simulink model "six_plus_six_AcmsteeringV09_main"  (R2014a)
settings: Solver=FixedStepDiscrete  StartTime=0.0  StopTime=10.0  FixedStep=0.0005  RelTol=1e-3
InitFcn:
  | Veh_Par_wxt
values from neighbouring files (symbols this model uses):
  acc_spdctl = [0 100]    [Veh_Par_wxt.m]
  ag_thr = ecucoder_cal(ag_thr)    [Veh_Par_wxt.m]
  B = 1.8    [Veh_Par_wxt.m]
  bra_em = 100    [Veh_Par_wxt.m]
  bra_pre_gz2 = 100/3    (= 33.3333333333)    [Veh_Par_wxt.m]
  bra_pre_gz34 = 10/3    (= 3.33333333333)    [Veh_Par_wxt.m]
  bra_pre_yd = 10/2    (= 5)    [Veh_Par_wxt.m]
  brakepre_dem_data = [0 1 2 3 4 5 6 7 8 9 10]    [Veh_Par_wxt.m]
  brakeTrq_dem_data = [0 125 251 376 502 627 753 878 1004 1129 1255]    [Veh_Par_wxt.m]
  bratrq_max = 4*1255    (= 5020)    [Veh_Par_wxt.m]
  eff_tran = 0.9    [Veh_Par_wxt.m]
  ESP_switch = ecucoder_cal(ESP_switch)    [Veh_Par_wxt.m]
  G = Mass*g    (= 15696)    [Veh_Par_wxt.m]
  kd1 = ecucoder_cal(kd1)    [Veh_Par_wxt.m]
  kd2 = 0    [Veh_Par_wxt.m]
  ki1 = ecucoder_cal(ki1)    [Veh_Par_wxt.m]
  ki2 = 1    [Veh_Par_wxt.m]
  kp1 = ecucoder_cal(kp1)    [Veh_Par_wxt.m]
  kp2 = 300    [Veh_Par_wxt.m]
  L = L1+L2    (= 2.9)    [Veh_Par_wxt.m]
  premax = 100    [Veh_Par_wxt.m]
  Radius = 0.4572/2    (= 0.2286)    [Veh_Par_wxt.m]
  RC_switch = ecucoder_cal(RC_switch)    [Veh_Par_wxt.m]
  s_opt_yi = 0.15    [Veh_Par_wxt.m]
  s_opt_zhuan = 0.8    [Veh_Par_wxt.m]
  s_opt_zhuan_add = 0.05    [Veh_Par_wxt.m]
  s_opt_zhuan_table = [0.8 0.8 0.3 0.3]    [Veh_Par_wxt.m]
  spd_map_mot = [0 499.85 999.79 1500 2000 2500 3000 3500 4000 4500 4999.8 5999.8]    [Veh_Par_wxt.m]
  spd_spdctl = [0 500]    [Veh_Par_wxt.m]
  speed_thr_park = 5/3.6/Radius*tras_ratio*30/pi    (= 464.143899364)    [Veh_Par_wxt.m]
  TCS_switch = ecucoder_cal(TCS_switch)    [Veh_Par_wxt.m]
  tras_ratio = 8    [Veh_Par_wxt.m]
  trq_map_mot = [70.5 70.012 71.154 65.797 53.917 45.159 38.073 32.685 27.48 17.133 14.949 10.07]    [Veh_Par_wxt.m]
  trqmax_yd = 70.5    [Veh_Par_wxt.m]
  trqmax_zx = 70.5    [Veh_Par_wxt.m]
  trqmaxneg = -70.5    [Veh_Par_wxt.m]
  v_gain = 0.9    [Veh_Par_wxt.m]
  v_table = [0 5 20 100]    [Veh_Par_wxt.m]
  v_thr_park = 5    [Veh_Par_wxt.m]
  zhidong_bianmazhi = [-140000 750000]    [Veh_Par_wxt.m]
  zhidong_down = -140000    [Veh_Par_wxt.m]
  zhidong_up = 750000    [Veh_Par_wxt.m]
  zhidong_youmen = [0 100]    [Veh_Par_wxt.m]
  zhuanxiang_bianmazhi = [-400000 0 400000]    [Veh_Par_wxt.m]
  zhuanxiang_down = -400000    [Veh_Par_wxt.m]
  zhuanxiang_up = 400000    [Veh_Par_wxt.m]
  zhuanxiang_youmen = [-100 0 100]    [Veh_Par_wxt.m]
undefined symbols (not defined in the file or in its folder): ecucoder_acal, guzhang_lf, guzhang_lm, guzhang_lr, guzhang_rf, guzhang_rm, guzhang_rr, myFIS
libraries: simulink x979, ec5744lib x59, fuzblock x2
(part 23 of 26)

== matlab function six_plus_six_AcmsteeringV09_main/MainControl/mode_control/backward/backward/Drive/容错控制/MATLAB Function ==
  data: trq_dem_l input; trq_dem_lf output; trq_dem_lm output; trq_dem_r input; trqlim_lf input; trqlim_lm input; trqlim_lr input; trqlim_rf input; trqlim_rm input; trqlim_rr input; guzhang_lf input; guzhang_lm input; guzhang_lr input; guzhang_rf input; guzhang_rm input; guzhang_rr input; trq_dem_lr output; trq_dem_rf output; trq_dem_rm output; trq_dem_rr output; bra_pre_l output; bra_pre_r output; bra_pre_gz2 input; bra_pre_gz34 input; mode output int8
function [trq_dem_lf,trq_dem_lm,trq_dem_lr,trq_dem_rf,trq_dem_rm,trq_dem_rr,bra_pre_l,bra_pre_r,mode] = fcn(trq_dem_l,trq_dem_r,trqlim_lf,trqlim_lm,trqlim_lr,trqlim_rf,trqlim_rm,trqlim_rr,guzhang_lf,guzhang_lm,guzhang_lr,guzhang_rf,guzhang_rm,guzhang_rr,bra_pre_gz2,bra_pre_gz34)
%#codegen
if guzhang_lf==0 && guzhang_lm==0 && guzhang_lr==0 && guzhang_rf==0 && guzhang_rm==0 && guzhang_rr==0    %0电机故障,平均分配
    trq_dem_lf=single(trq_dem_l/3);
    trq_dem_lm=single(trq_dem_l/3);
    trq_dem_lr=single(trq_dem_l/3);
    trq_dem_rf=single(trq_dem_r/3);
    trq_dem_rm=single(trq_dem_r/3);
    trq_dem_rr=single(trq_dem_r/3);
    bra_pre_l=single(0);
    bra_pre_r=single(0);
    mode=int8(1);
    
    
    
    
elseif guzhang_lf==1 && guzhang_lm==0 && guzhang_lr==0 && guzhang_rf==0 && guzhang_rm==0 && guzhang_rr==0    %1电机故障，同侧电机进行力矩转移，超过限值后，对侧亦降扭。  左前
    trq_dem_lf=single(0);
    trq_dem_lm=single(min(trq_dem_l/2,trqlim_lm));
    trq_dem_lr=single(min(trq_dem_l/2,trqlim_lr));
    trq_dem_rf=single((trq_dem_r-(trq_dem_l-trq_dem_lm-trq_dem_lr))/3);
    trq_dem_rm=single((trq_dem_r-(trq_dem_l-trq_dem_lm-trq_dem_lr))/3);
    trq_dem_rr=single((trq_dem_r-(trq_dem_l-trq_dem_lm-trq_dem_lr))/3);
    bra_pre_l=single(0);
    bra_pre_r=single(0);
    mode=int8(2);
elseif guzhang_lf==0 && guzhang_lm==1 && guzhang_lr==0 && guzhang_rf==0 && guzhang_rm==0 && guzhang_rr==0    %1电机故障，同侧电机进行力矩转移，超过限值后，对侧亦降扭。 左中
    trq_dem_lf=single(min(trq_dem_l/2,trqlim_lf));
    trq_dem_lm=single(0);
    trq_dem_lr=single(min(trq_dem_l/2,trqlim_lr));
    trq_dem_rf=single((trq_dem_r-(trq_dem_l-trq_dem_lf-trq_dem_lr))/3);
    trq_dem_rm=single((trq_dem_r-(trq_dem_l-trq_dem_lf-trq_dem_lr))/3);
    trq_dem_rr=single((trq_dem_r-(trq_dem_l-trq_dem_lf-trq_dem_lr))/3);
    bra_pre_l=single(0);
    bra_pre_r=single(0);
    mode=int8(3);
elseif guzhang_lf==0 && guzhang_lm==0 && guzhang_lr==1 && guzhang_rf==0 && guzhang_rm==0 && guzhang_rr==0    %1电机故障，同侧电机进行力矩转移，超过限值后，对侧亦降扭。 左后
    trq_dem_lf=single(min(trq_dem_l/2,trqlim_lf));
    trq_dem_lm=single(min(trq_dem_l/2,trqlim_lm));
    trq_dem_lr=single(0);
    trq_dem_rf=single((trq_dem_r-(trq_dem_l-trq_dem_lf-trq_dem_lm))/3);
    trq_dem_rm=single((trq_dem_r-(trq_dem_l-trq_dem_lf-trq_dem_lm))/3);
    trq_dem_rr=single((trq_dem_r-(trq_dem_l-trq_dem_lf-trq_dem_lm))/3);
    bra_pre_l=single(0);
    bra_pre_r=single(0);
    mode=int8(4);
elseif guzhang_lf==0 && guzhang_lm==0 && guzhang_lr==0 && guzhang_rf==1 && guzhang_rm==0 && guzhang_rr==0    %1电机故障，同侧电机进行力矩转移，超过限值后，对侧亦降扭。  右前
    trq_dem_rf=single(0);
    trq_dem_rm=single(min(trq_dem_r/2,trqlim_rm));
    trq_dem_rr=single(min(trq_dem_r/2,trqlim_rr));
    trq_dem_lf=single((trq_dem_l-(trq_dem_r-trq_dem_rm-trq_dem_rr))/3);
    trq_dem_lm=single((trq_dem_l-(trq_dem_r-trq_dem_rm-trq_dem_rr))/3);
    trq_dem_lr=single((trq_dem_l-(trq_dem_r-trq_dem_rm-trq_dem_rr))/3);
    bra_pre_l=single(0);
    bra_pre_r=single(0);
    mode=int8(5);
elseif guzhang_lf==0 && guzhang_lm==0 && guzhang_lr==0 && guzhang_rf==0 && guzhang_rm==1 && guzhang_rr==0    %1电机故障，同侧电机进行力矩转移，超过限值后，对侧亦降扭。 右中
    trq_dem_rf=single(min(trq_dem_r/2,trqlim_rf));
    trq_dem_rm=single(0);
    trq_dem_rr=single(min(trq_dem_r/2,trqlim_rr));
    trq_dem_lf=single((trq_dem_l-(trq_dem_r-trq_dem_rf-trq_dem_rr))/3);
    trq_dem_lm=single((trq_dem_l-(trq_dem_r-trq_dem_rf-trq_dem_rr))/3);
    trq_dem_lr=single((trq_dem_l-(trq_dem_r-trq_dem_rf-trq_dem_rr))/3);
    bra_pre_l=single(0);
    bra_pre_r=single(0);
    mode=int8(6);
elseif guzhang_lf==0 && guzhang_lm==0 && guzhang_lr==0 && guzhang_rf==0 && guzhang_rm==0 && guzhang_rr==1    %1电机故障，同侧电机进行力矩转移，超过限值后，对侧亦降扭。 右后
    trq_dem_rf=single(min(trq_dem_r/2,trqlim_rf));
    trq_dem_rm=single(min(trq_dem_r/2,trqlim_rm));
    trq_dem_rr=single(0);
    trq_dem_lf=single((trq_dem_l-(trq_dem_r-trq_dem_rf-trq_dem_rm))/3);
    trq_dem_lm=single((trq_dem_l-(trq_dem_r-trq_dem_rf-trq_dem_rm))/3);
    trq_dem_lr=single((trq_dem_l-(trq_dem_r-trq_dem_rf-trq_dem_rm))/3);
    bra_pre_l=single(0);
    bra_pre_r=single(0);
    mode=int8(7);
    
    
    
    
    
    
elseif guzhang_lf==1 && guzhang_lm==1 && guzhang_lr==0 && guzhang_rf==0 && guzhang_rm==0 && guzhang_rr==0    %2电机故障，同侧电机进行力矩转移，超过限值后，对侧亦降扭。  左前 左中   左侧
    trq_dem_lf=single(0);
    trq_dem_lm=single(0);
    trq_dem_lr=single(min(trq_dem_l,trqlim_lr));
    trq_dem_rf=single((trq_dem_r-(trq_dem_l-trq_dem_lr))/3);
    trq_dem_rm=single((trq_dem_r-(trq_dem_l-trq_dem_lr))/3);
    trq_dem_rr=single((trq_dem_r-(trq_dem_l-trq_dem_lr))/3);
    bra_pre_l=single(0);
    bra_pre_r=single(0);
    mode=int8(8);
elseif guzhang_lf==1 && guzhang_lm==0 && guzhang_lr==1 && guzhang_rf==0 && guzhang_rm==0 && guzhang_rr==0    %2电机故障，同侧电机进行力矩转移，超过限值后，对侧亦降扭。  左前 左后
    trq_dem_lf=single(0);
    trq_dem_lm=single(min(trq_dem_l,trqlim_lm));
    trq_dem_lr=single(0);
    trq_dem_rf=single((trq_dem_r-(trq_dem_l-trq_dem_lm))/3);
    trq_dem_rm=single((trq_dem_r-(trq_dem_l-trq_dem_lm))/3);
    trq_dem_rr=single((trq_dem_r-(trq_dem_l-trq_dem_lm))/3);
    bra_pre_l=single(0);
    bra_pre_r=single(0);
    mode=int8(9);
elseif guzhang_lf==0 && guzhang_lm==1 && guzhang_lr==1 && guzhang_rf==0 && guzhang_rm==0 && guzhang_rr==0    %2电机故障，同侧电机进行力矩转移，超过限值后，对侧亦降扭。  左中 左后
    trq_dem_lf=single(min(trq_dem_l,trqlim_lf));
    trq_dem_lm=single(0);
    trq_dem_lr=single(0);
    trq_dem_rf=single((trq_dem_r-(trq_dem_l-trq_dem_lf))/3);
    trq_dem_rm=single((trq_dem_r-(trq_dem_l-trq_dem_lf))/3);
    trq_dem_rr=single((trq_dem_r-(trq_dem_l-trq_dem_lf))/3);
    bra_pre_l=single(0);
    bra_pre_r=single(0);
    mode=int8(10);
    
elseif guzhang_lf==0 && guzhang_lm==0 && guzhang_lr==0 && guzhang_rf==1 && guzhang_rm==1 && guzhang_rr==0    %2电机故障，同侧电机进行力矩转移，超过限值后，对侧亦降扭。  右前 右中   右侧
    trq_dem_rf=single(0);
    trq_dem_rm=single(0);
    trq_dem_rr=single(min(trq_dem_r,trqlim_rr));
    trq_dem_lf=single((trq_dem_l-(trq_dem_r-trq_dem_rr))/3);
    trq_dem_lm=single((trq_dem_l-(trq_dem_r-trq_dem_rr))/3);
    trq_dem_lr=single((trq_dem_l-(trq_dem_r-trq_dem_rr))/3);
    bra_pre_l=single(0);
    bra_pre_r=single(0);
    mode=int8(11);
elseif guzhang_lf==0 && guzhang_lm==0 && guzhang_lr==0 && guzhang_rf==1 && guzhang_rm==0 && guzhang_rr==1    %2电机故障，同侧电机进行力矩转移，超过限值后，对侧亦降扭。  右前 右后
    trq_dem_rf=single(0);
    trq_dem_rm=single(min(trq_dem_r,trqlim_rm));
    trq_dem_rr=single(0);
    trq_dem_lf=single((trq_dem_l-(trq_dem_r-trq_dem_rm))/3);
    trq_dem_lm=single((trq_dem_l-(trq_dem_r-trq_dem_rm))/3);
    trq_dem_lr=single((trq_dem_l-(trq_dem_r-trq_dem_rm))/3);
    bra_pre_l=single(0);
    bra_pre_r=single(0);
    mode=int8(12);
elseif guzhang_lf==0 && guzhang_lm==0 && guzhang_lr==0 && guzhang_rf==0 && guzhang_rm==1 && guzhang_rr==1    %2电机故障，同侧电机进行力矩转移，超过限值后，对侧亦降扭。  右中 右后
    trq_dem_rf=single(min(trq_dem_r,trqlim_rf));
    trq_dem_rm=single(0);
    trq_dem_rr=single(0);
    trq_dem_lf=single((trq_dem_l-(trq_dem_r-trq_dem_rf))/3);
    trq_dem_lm=single((trq_dem_l-(trq_dem_r-trq_dem_rf))/3);
    trq_dem_lr=single((trq_dem_l-(trq_dem_r-trq_dem_rf))/3);
    bra_pre_l=single(0);
    bra_pre_r=single(0);
    mode=int8(13);
    
elseif guzhang_lf==1 && guzhang_lm==0 && guzhang_lr==0 && guzhang_rf==1 && guzhang_rm==0 && guzhang_rr==0    %2电机故障，同侧电机进行力矩转移，超过限值后，对侧亦降扭。  左前-右前 对侧
    trq_dem_lf=single(0);
    trq_dem_rf=single(0);
    trq_dem_lm=single(min(trq_dem_l/2,trqlim_lm));
    trq_dem_lr=single(min(trq_dem_l/2,trqlim_lr));
    trq_dem_rm=single(min(trq_dem_r/2,trqlim_rm));
    trq_dem_rr=single(min(trq_dem_r/2,trqlim_rr));
    if (trq_dem_l-trq_dem_lm-trq_dem_lr)>=(trq_dem_r-trq_dem_rm-trq_dem_rr)
        trq_dem_rm=single(min(trqlim_rm,(trq_dem_r-(trq_dem_l-trq_dem_lm-trq_dem_lr))/2));
        trq_dem_rr=single(min(trqlim_rr,(trq_dem_r-(trq_dem_l-trq_dem_lm-trq_dem_lr))/2));
    else
        trq_dem_lm=single(min(trqlim_lm,(trq_dem_l-(trq_dem_r-trq_dem_rm-trq_dem_rr))/2));
        trq_dem_lr=single(min(trqlim_lr,(trq_dem_l-(trq_dem_r-trq_dem_rm-trq_dem_rr))/2));
    end
    bra_pre_l=single(0);
    bra_pre_r=single(0);
    mode=int8(14);
elseif guzhang_lf==1 && guzhang_lm==0 && guzhang_lr==0 && guzhang_rf==0 && guzhang_rm==1 && guzhang_rr==0    %2电机故障，同侧电机进行力矩转移，超过限值后，对侧亦降扭。  左前-右中
    trq_dem_lf=single(0);
    trq_dem_rm=single(0);
    trq_dem_lm=single(min(trq_dem_l/2,trqlim_lm));
    trq_dem_lr=single(min(trq_dem_l/2,trqlim_lr));
    trq_dem_rf=single(min(trq_dem_r/2,trqlim_rf));
    trq_dem_rr=single(min(trq_dem_r/2,trqlim_rr));
    if (trq_dem_l-trq_dem_lm-trq_dem_lr)>=(trq_dem_r-trq_dem_rf-trq_dem_rr)
        trq_dem_rf=single(min(trqlim_rf,(trq_dem_r-(trq_dem_l-trq_dem_lm-trq_dem_lr))/2));
        trq_dem_rr=single(min(trqlim_rr,(trq_dem_r-(trq_dem_l-trq_dem_lm-trq_dem_lr))/2));
    else
        trq_dem_lm=single(min(trqlim_lm,(trq_dem_l-(trq_dem_r-trq_dem_rf-trq_dem_rr))/2));
        trq_dem_lr=single(min(trqlim_lr,(trq_dem_l-(trq_dem_r-trq_dem_rf-trq_dem_rr))/2));
    end
    bra_pre_l=single(0);
    bra_pre_r=single(0);
    mode=int8(15);
elseif guzhang_lf==1 && guzhang_lm==0 && guzhang_lr==0 && guzhang_rf==0 && guzhang_rm==0 && guzhang_rr==1    %2电机故障，同侧电机进行力矩转移，超过限值后，对侧亦降扭。  左前-右后
    trq_dem_lf=single(0);
    trq_dem_rr=single(0);
    trq_dem_lm=single(min(trq_dem_l/2,trqlim_lm));
    trq_dem_lr=single(min(trq_dem_l/2,trqlim_lr));
    trq_dem_rf=single(min(trq_dem_r/2,trqlim_rf));
    trq_dem_rm=single(min(trq_dem_r/2,trqlim_rm));
    if (trq_dem_l-trq_dem_lm-trq_dem_lr)>=(trq_dem_r-trq_dem_rf-trq_dem_rm)
        trq_dem_rf=single(min(trqlim_rf,(trq_dem_r-(trq_dem_l-trq_dem_lm-trq_dem_lr))/2));
        trq_dem_rm=single(min(trqlim_rm,(trq_dem_r-(trq_dem_l-trq_dem_lm-trq_dem_lr))/2));
    else
        trq_dem_lm=single(min(trqlim_lm,(trq_dem_l-(trq_dem_r-trq_dem_rf-trq_dem_rm))/2));
        trq_dem_lr=single(min(trqlim_lr,(trq_dem_l-(trq_dem_r-trq_dem_rf-trq_dem_rm))/2));
    end
    bra_pre_l=single(0);
    bra_pre_r=single(0);
    mode=int8(16);
    
elseif guzhang_lf==0 && guzhang_lm==1 && guzhang_lr==0 && guzhang_rf==1 && guzhang_rm==0 && guzhang_rr==0    %2电机故障，同侧电机进行力矩转移，超过限值后，对侧亦降扭。  左中-右前
    trq_dem_lm=single(0);
    trq_dem_rf=single(0);
    trq_dem_lf=single(min(trq_dem_l/2,trqlim_lf));
    trq_dem_lr=single(min(trq_dem_l/2,trqlim_lr));
    trq_dem_rm=single(min(trq_dem_r/2,trqlim_rm));
    trq_dem_rr=single(min(trq_dem_r/2,trqlim_rr));
    if (trq_dem_l-trq_dem_lf-trq_dem_lr)>=(trq_dem_r-trq_dem_rm-trq_dem_rr)
        trq_dem_rm=single(min(trqlim_rm,(trq_dem_r-(trq_dem_l-trq_dem_lf-trq_dem_lr))/2));
        trq_dem_rr=single(min(trqlim_rr,(trq_dem_r-(trq_dem_l-trq_dem_lf-trq_dem_lr))/2));
    else
        trq_dem_lf=single(min(trqlim_lf,(trq_dem_l-(trq_dem_r-trq_dem_rm-trq_dem_rr))/2));
        trq_dem_lr=single(min(trqlim_lr,(trq_dem_l-(trq_dem_r-trq_dem_rm-trq_dem_rr))/2));
    end
    bra_pre_l=single(0);
    bra_pre_r=single(0);
    mode=int8(17);
elseif guzhang_lf==0 && guzhang_lm==1 && guzhang_lr==0 && guzhang_rf==0 && guzhang_rm==1 && guzhang_rr==0    %2电机故障，同侧电机进行力矩转移，超过限值后，对侧亦降扭。  左中-右中
    trq_dem_lm=single(0);
    trq_dem_rm=single(0);
    trq_dem_lf=single(min(trq_dem_l/2,trqlim_lf));
    trq_dem_lr=single(min(trq_dem_l/2,trqlim_lr));
    trq_dem_rf=single(min(trq_dem_r/2,trqlim_rf));
    trq_dem_rr=single(min(trq_dem_r/2,trqlim_rr));
    if (trq_dem_l-trq_dem_lf-trq_dem_lr)>=(trq_dem_r-trq_dem_rf-trq_dem_rr)
        trq_dem_rf=single(min(trqlim_rf,(trq_dem_r-(trq_dem_l-trq_dem_lf-trq_dem_lr))/2));
        trq_dem_rr=single(min(trqlim_rr,(trq_dem_r-(trq_dem_l-trq_dem_lf-trq_dem_lr))/2));
    else
        trq_dem_lf=single(min(trqlim_lf,(trq_dem_l-(trq_dem_r-trq_dem_rf-trq_dem_rr))/2));
        trq_dem_lr=single(min(trqlim_lr,(trq_dem_l-(trq_dem_r-trq_dem_rf-trq_dem_rr))/2));
    end
    bra_pre_l=single(0);
    bra_pre_r=single(0);
    mode=int8(18);
elseif guzhang_lf==0 && guzhang_lm==1 && guzhang_lr==0 && guzhang_rf==0 && guzhang_rm==0 && guzhang_rr==1    %2电机故障，同侧电机进行力矩转移，超过限值后，对侧亦降扭。  左中-右后
    trq_dem_lm=single(0);
    trq_dem_rr=single(0);
    trq_dem_lf=single(min(trq_dem_l/2,trqlim_lf));
    trq_dem_lr=single(min(trq_dem_l/2,trqlim_lr));
    trq_dem_rf=single(min(trq_dem_r/2,trqlim_rf));
    trq_dem_rm=single(min(trq_dem_r/2,trqlim_rm));
    if (trq_dem_l-trq_dem_lf-trq_dem_lr)>=(trq_dem_r-trq_dem_rf-trq_dem_rm)
        trq_dem_rf=single(min(trqlim_rf,(trq_dem_r-(trq_dem_l-trq_dem_lf-trq_dem_lr))/2));
        trq_dem_rm=single(min(trqlim_rm,(trq_dem_r-(trq_dem_l-trq_dem_lf-trq_dem_lr))/2));
    else
        trq_dem_lf=single(min(trqlim_lf,(trq_dem_l-(trq_dem_r-trq_dem_rf-trq_dem_rm))/2));
        trq_dem_lr=single(min(trqlim_lr,(trq_dem_l-(trq_dem_r-trq_dem_rf-trq_dem_rm))/2));
    end
    bra_pre_l=single(0);
    bra_pre_r=single(0);
    mode=int8(19);
    
elseif guzhang_lf==0 && guzhang_lm==0 && guzhang_lr==1 && guzhang_rf==1 && guzhang_rm==0 && guzhang_rr==0    %2电机故障，同侧电机进行力矩转移，超过限值后，对侧亦降扭。  左后-右前
    trq_dem_lr=single(0);
    trq_dem_rf=single(0);
    trq_dem_lf=single(min(trq_dem_l/2,trqlim_lf));
    trq_dem_lm=single(min(trq_dem_l/2,trqlim_lm));
    trq_dem_rm=single(min(trq_dem_r/2,trqlim_rm));
    trq_dem_rr=single(min(trq_dem_r/2,trqlim_rr));
    if (trq_dem_l-trq_dem_lf-trq_dem_lm)>=(trq_dem_r-trq_dem_rm-trq_dem_rr)
        trq_dem_rm=single(min(trqlim_rm,(trq_dem_r-(trq_dem_l-trq_dem_lf-trq_dem_lm))/2));
        trq_dem_rr=single(min(trqlim_rr,(trq_dem_r-(trq_dem_l-trq_dem_lf-trq_dem_lm))/2));
    else
        trq_dem_lf=single(min(trqlim_lf,(trq_dem_l-(trq_dem_r-trq_dem_rm-trq_dem_rr))/2));
        trq_dem_lm=single(min(trqlim_lm,(trq_dem_l-(trq_dem_r-trq_dem_rm-trq_dem_rr))/2));
    end
    bra_pre_l=single(0);
    bra_pre_r=single(0);
    mode=int8(20);
elseif guzhang_lf==0 && guzhang_lm==0 && guzhang_lr==1 && guzhang_rf==0 && guzhang_rm==1 && guzhang_rr==0    %2电机故障，同侧电机进行力矩转移，超过限值后，对侧亦降扭。  左后-右中
    trq_dem_lr=single(0);
    trq_dem_rm=single(0);
    trq_dem_lf=single(min(trq_dem_l/2,trqlim_lf));
    trq_dem_lm=single(min(trq_dem_l/2,trqlim_lm));
    trq_dem_rf=single(min(trq_dem_r/2,trqlim_rf));
    trq_dem_rr=single(min(trq_dem_r/2,trqlim_rr));
    if (trq_dem_l-trq_dem_lf-trq_dem_lm)>=(trq_dem_r-trq_dem_rf-trq_dem_rr)
        trq_dem_rf=single(min(trqlim_rf,(trq_dem_r-(trq_dem_l-trq_dem_lf-trq_dem_lm))/2));
        trq_dem_rr=single(min(trqlim_rr,(trq_dem_r-(trq_dem_l-trq_dem_lf-trq_dem_lm))/2));
    else
        trq_dem_lf=single(min(trqlim_lf,(trq_dem_l-(trq_dem_r-trq_dem_rf-trq_dem_rr))/2));
        trq_dem_lm=single(min(trqlim_lm,(trq_dem_l-(trq_dem_r-trq_dem_rf-trq_dem_rr))/2));
    end
    bra_pre_l=single(0);
    bra_pre_r=single(0);
    mode=int8(21);
elseif guzhang_lf==0 && guzhang_lm==0 && guzhang_lr==1 && guzhang_rf==0 && guzhang_rm==0 && guzhang_rr==1    %2电机故障，同侧电机进行力矩转移，超过限值后，对侧亦降扭。  左后-右后
    trq_dem_lr=single(0);
    trq_dem_rr=single(0);
    trq_dem_lf=single(min(trq_dem_l/2,trqlim_lf));
    trq_dem_lm=single(min(trq_dem_l/2,trqlim_lm));
    trq_dem_rf=single(min(trq_dem_r/2,trqlim_rf));
    trq_dem_rm=single(min(trq_dem_r/2,trqlim_rm));
    if (trq_dem_l-trq_dem_lf-trq_dem_lm)>=(trq_dem_r-trq_dem_rf-trq_dem_rm)
        trq_dem_rf=single(min(trqlim_rf,(trq_dem_r-(trq_dem_l-trq_dem_lf-trq_dem_lm))/2));
        trq_dem_rm=single(min(trqlim_rm,(trq_dem_r-(trq_dem_l-trq_dem_lf-trq_dem_lm))/2));
    else
        trq_dem_lf=single(min(trqlim_lf,(trq_dem_l-(trq_dem_r-trq_dem_rf-trq_dem_rm))/2));
        trq_dem_lm=single(min(trqlim_lm,(trq_dem_l-(trq_dem_r-trq_dem_rf-trq_dem_rm))/2));
    end
    bra_pre_l=single(0);
    bra_pre_r=single(0);
    mode=int8(22);
    
    
    
    
    
    
    
    
    
elseif guzhang_lf==1 && guzhang_lm==1 && guzhang_lr==1 && guzhang_rf==0 && guzhang_rm==0 && guzhang_rr==0    %3电机故障，同侧电机进行力矩转移，超过限值后，对侧亦降扭。  左前 左中 左后   左侧
    trq_dem_lf=single(0);
    trq_dem_lm=single(0);
    trq_dem_lr=single(0);
    trq_dem_rf=single(0);
    trq_dem_rm=single(0);
    trq_dem_rr=single(0);
    bra_pre_l=single(bra_pre_gz2);
    bra_pre_r=single(bra_pre_gz2);
    mode=int8(23);
elseif guzhang_lf==0 && guzhang_lm==0 && guzhang_lr==0 && guzhang_rf==1 && guzhang_rm==1 && guzhang_rr==1    %3电机故障，同侧电机进行力矩转移，超过限值后，对侧亦降扭。  右前 右中 右后   右侧
    trq_dem_lf=single(0);
    trq_dem_lm=single(0);
    trq_dem_lr=single(0);
    trq_dem_rf=single(0);
    trq_dem_rm=single(0);
    trq_dem_rr=single(0);
    bra_pre_l=single(bra_pre_gz2);
    bra_pre_r=single(bra_pre_gz2);
    mode=int8(24);
    
elseif guzhang_lf==1 && guzhang_lm==1 && guzhang_lr==0 && guzhang_rf==1 && guzhang_rm==0 && guzhang_rr==0    %3电机故障，同侧电机进行力矩转移，超过限值后，对侧亦降扭。  左前-左中-右前 对侧
    trq_dem_lf=single(0);
    trq_dem_lm=single(0);
    trq_dem_rf=single(0);
    trq_dem_lr=single(min(trq_dem_l,trqlim_lr));
    trq_dem_rm=single(min(trq_dem_r/2,trqlim_rm));
    trq_dem_rr=single(min(trq_dem_r/2,trqlim_rr));
    if (trq_dem_l-trq_dem_lr)>=(trq_dem_r-trq_dem_rm-trq_dem_rr)
        trq_dem_rm=single(min(trqlim_rm,(trq_dem_r-(trq_dem_l-trq_dem_lr))/2));
        trq_dem_rr=single(min(trqlim_rr,(trq_dem_r-(trq_dem_l-trq_dem_lr))/2));
    else
        trq_dem_lr=single(min(trqlim_lr,(trq_dem_l-(trq_dem_r-trq_dem_rm-trq_dem_rr))));
    end
    bra_pre_l=single(0);
    bra_pre_r=single(0);
    mode=int8(25);
elseif guzhang_lf==1 && guzhang_lm==1 && guzhang_lr==0 && guzhang_rf==0 && guzhang_rm==1 && guzhang_rr==0    %3电机故障，同侧电机进行力矩转移，超过限值后，对侧亦降扭。  左前-左中-右中 对侧
    trq_dem_lf=single(0);
    trq_dem_lm=single(0);
    trq_dem_rm=single(0);
    trq_dem_lr=single(min(trq_dem_l,trqlim_lr));
    trq_dem_rf=single(min(trq_dem_r/2,trqlim_rf));
    trq_dem_rr=single(min(trq_dem_r/2,trqlim_rr));
    if (trq_dem_l-trq_dem_lr)>=(trq_dem_r-trq_dem_rf-trq_dem_rr)
        trq_dem_rf=single(min(trqlim_rf,(trq_dem_r-(trq_dem_l-trq_dem_lr))/2));
        trq_dem_rr=single(min(trqlim_rr,(trq_dem_r-(trq_dem_l-trq_dem_lr))/2));
    else
        trq_dem_lr=single(min(trqlim_lr,(trq_dem_l-(trq_dem_r-trq_dem_rf-trq_dem_rr))));
    end
    bra_pre_l=single(0);
    bra_pre_r=single(0);
    mode=int8(26);
elseif guzhang_lf==1 && guzhang_lm==1 && guzhang_lr==0 && guzhang_rf==0 && guzhang_rm==0 && guzhang_rr==1    %3电机故障，同侧电机进行力矩转移，超过限值后，对侧亦降扭。  左前-左中-右后 对侧
    trq_dem_lf=single(0);
    trq_dem_lm=single(0);
    trq_dem_rr=single(0);
    trq_dem_lr=single(min(trq_dem_l,trqlim_lr));
    trq_dem_rf=single(min(trq_dem_r/2,trqlim_rf));
    trq_dem_rm=single(min(trq_dem_r/2,trqlim_rm));
    if (trq_dem_l-trq_dem_lr)>=(trq_dem_r-trq_dem_rf-trq_dem_rm)
        trq_dem_rf=single(min(trqlim_rf,(trq_dem_r-(trq_dem_l-trq_dem_lr))/2));
        trq_dem_rm=single(min(trqlim_rm,(trq_dem_r-(trq_dem_l-trq_dem_lr))/2));
    else
        trq_dem_lr=single(min(trqlim_lr,(trq_dem_l-(trq_dem_r-trq_dem_rf-trq_dem_rm))));
    end
    bra_pre_l=single(0);
    bra_pre_r=single(0);
    mode=int8(27);
    
elseif guzhang_lf==1 && guzhang_lm==0 && guzhang_lr==1 && guzhang_rf==1 && guzhang_rm==0 && guzhang_rr==0    %3电机故障，同侧电机进行力矩转移，超过限值后，对侧亦降扭。  左前-左后-右前 对侧
    trq_dem_lf=single(0);
    trq_dem_lr=single(0);
    trq_dem_rf=single(0);
    trq_dem_lm=single(min(trq_dem_l,trqlim_lm));
    trq_dem_rm=single(min(trq_dem_r/2,trqlim_rm));
    trq_dem_rr=single(min(trq_dem_r/2,trqlim_rr));
    if (trq_dem_l-trq_dem_lm)>=(trq_dem_r-trq_dem_rm-trq_dem_rr)
        trq_dem_rm=single(min(trqlim_rm,(trq_dem_r-(trq_dem_l-trq_dem_lm))/2));
        trq_dem_rr=single(min(trqlim_rr,(trq_dem_r-(trq_dem_l-trq_dem_lm))/2));
    else
        trq_dem_lm=single(min(trqlim_lm,(trq_dem_l-(trq_dem_r-trq_dem_rm-trq_dem_rr))));
    end
    bra_pre_l=single(0);
    bra_pre_r=single(0);
    mode=int8(28);
elseif guzhang_lf==1 && guzhang_lm==0 && guzhang_lr==1 && guzhang_rf==0 && guzhang_rm==1 && guzhang_rr==0    %3电机故障，同侧电机进行力矩转移，超过限值后，对侧亦降扭。  左前-左后-右中 对侧
    trq_dem_lf=single(0);
    trq_dem_lr=single(0);
    trq_dem_rm=single(0);
    trq_dem_lm=single(min(trq_dem_l,trqlim_lm));
    trq_dem_rf=single(min(trq_dem_r/2,trqlim_rf));
    trq_dem_rr=single(min(trq_dem_r/2,trqlim_rr));
    if (trq_dem_l-trq_dem_lm)>=(trq_dem_r-trq_dem_rf-trq_dem_rr)
        trq_dem_rf=single(min(trqlim_rf,(trq_dem_r-(trq_dem_l-trq_dem_lm))/2));
        trq_dem_rr=single(min(trqlim_rr,(trq_dem_r-(trq_dem_l-trq_dem_lm))/2));
    else
        trq_dem_lm=single(min(trqlim_lm,(trq_dem_l-(trq_dem_r-trq_dem_rf-trq_dem_rr))));
    end
    bra_pre_l=single(0);
    bra_pre_r=single(0);
    mode=int8(29);
elseif guzhang_lf==1 && guzhang_lm==0 && guzhang_lr==1 && guzhang_rf==0 && guzhang_rm==0 && guzhang_rr==1    %3电机故障，同侧电机进行力矩转移，超过限值后，对侧亦降扭。  左前-左后-右后 对侧
    trq_dem_lf=single(0);
    trq_dem_lr=single(0);
    trq_dem_rr=single(0);
    trq_dem_lm=single(min(trq_dem_l,trqlim_lm));
    trq_dem_rf=single(min(trq_dem_r/2,trqlim_rf));
    trq_dem_rm=single(min(trq_dem_r/2,trqlim_rm));
    if (trq_dem_l-trq_dem_lm)>=(trq_dem_r-trq_dem_rf-trq_dem_rm)
        trq_dem_rf=single(min(trqlim_rf,(trq_dem_r-(trq_dem_l-trq_dem_lm))/2));
        trq_dem_rm=single(min(trqlim_rm,(trq_dem_r-(trq_dem_l-trq_dem_lm))/2));
    else
        trq_dem_lm=single(min(trqlim_lm,(trq_dem_l-(trq_dem_r-trq_dem_rf-trq_dem_rm))));
    end
    bra_pre_l=single(0);
    bra_pre_r=single(0);
    mode=int8(30);
    
elseif guzhang_lf==0 && guzhang_lm==1 && guzhang_lr==1 && guzhang_rf==1 && guzhang_rm==0 && guzhang_rr==0    %3电机故障，同侧电机进行力矩转移，超过限值后，对侧亦降扭。  左中-左后-右前 对侧
    trq_dem_lm=single(0);
    trq_dem_lr=single(0);
    trq_dem_rf=single(0);
    trq_dem_lf=single(min(trq_dem_l,trqlim_lf));
    trq_dem_rm=single(min(trq_dem_r/2,trqlim_rm));
    trq_dem_rr=single(min(trq_dem_r/2,trqlim_rr));
    if (trq_dem_l-trq_dem_lf)>=(trq_dem_r-trq_dem_rm-trq_dem_rr)
        trq_dem_rm=single(min(trqlim_rm,(trq_dem_r-(trq_dem_l-trq_dem_lf))/2));
        trq_dem_rr=single(min(trqlim_rr,(trq_dem_r-(trq_dem_l-trq_dem_lf))/2));
    else
        trq_dem_lf=single(min(trqlim_lf,(trq_dem_l-(trq_dem_r-trq_dem_rm-trq_dem_rr))));
    end
    bra_pre_l=single(0);
    bra_pre_r=single(0);
    mode=int8(31);
elseif guzhang_lf==0 && guzhang_lm==1 && guzhang_lr==1 && guzhang_rf==0 && guzhang_rm==1 && guzhang_rr==0    %3电机故障，同侧电机进行力矩转移，超过限值后，对侧亦降扭。  左中-左后-右中 对侧
    trq_dem_lm=single(0);
    trq_dem_lr=single(0);
    trq_dem_rm=single(0);
    trq_dem_lf=single(min(trq_dem_l,trqlim_lf));
    trq_dem_rf=single(min(trq_dem_r/2,trqlim_rf));
    trq_dem_rr=single(min(trq_dem_r/2,trqlim_rr));
    if (trq_dem_l-trq_dem_lf)>=(trq_dem_r-trq_dem_rf-trq_dem_rr)
        trq_dem_rf=single(min(trqlim_rf,(trq_dem_r-(trq_dem_l-trq_dem_lf))/2));
        trq_dem_rr=single(min(trqlim_rr,(trq_dem_r-(trq_dem_l-trq_dem_lf))/2));
    else
        trq_dem_lf=single(min(trqlim_lf,(trq_dem_l-(trq_dem_r-trq_dem_rf-trq_dem_rr))));
    end
    bra_pre_l=single(0);
    bra_pre_r=single(0);
    mode=int8(32);
elseif guzhang_lf==0 && guzhang_lm==1 && guzhang_lr==1 && guzhang_rf==0 && guzhang_rm==0 && guzhang_rr==1    %3电机故障，同侧电机进行力矩转移，超过限值后，对侧亦降扭。  左中-左后-右后 对侧
    trq_dem_lm=single(0);
    trq_dem_lr=single(0);
    trq_dem_rr=single(0);
    trq_dem_lf=single(min(trq_dem_l,trqlim_lf));
    trq_dem_rf=single(min(trq_dem_r/2,trqlim_rf));
    trq_dem_rm=single(min(trq_dem_r/2,trqlim_rm));
    if (trq_dem_l-trq_dem_lf)>=(trq_dem_r-trq_dem_rf-trq_dem_rm)
        trq_dem_rf=single(min(trqlim_rf,(trq_dem_r-(trq_dem_l-trq_dem_lf))/2));
        trq_dem_rm=single(min(trqlim_rm,(trq_dem_r-(trq_dem_l-trq_dem_lf))/2));
    else
        trq_dem_lf=single(min(trqlim_lf,(trq_dem_l-(trq_dem_r-trq_dem_rf-trq_dem_rm))));
    end
    bra_pre_l=single(0);
    bra_pre_r=single(0);
    mode=int8(33);
    
elseif guzhang_lf==1 && guzhang_lm==0 && guzhang_lr==0 && guzhang_rf==1 && guzhang_rm==1 && guzhang_rr==0    %3电机故障，同侧电机进行力矩转移，超过限值后，对侧亦降扭。  右前-右中-左前 对侧
    trq_dem_rf=single(0);
    trq_dem_rm=single(0);
    trq_dem_lf=single(0);
    trq_dem_rr=single(min(trq_dem_r,trqlim_rr));
    trq_dem_lm=single(min(trq_dem_l/2,trqlim_lm));
    trq_dem_lr=single(min(trq_dem_l/2,trqlim_lr));
    if (trq_dem_r-trq_dem_rr)>=(trq_dem_l-trq_dem_lm-trq_dem_lr)
        trq_dem_lm=single(min(trqlim_lm,(trq_dem_l-(trq_dem_r-trq_dem_rr))/2));
        trq_dem_lr=single(min(trqlim_lr,(trq_dem_l-(trq_dem_r-trq_dem_rr))/2));
    else
        trq_dem_rr=single(min(trqlim_rr,(trq_dem_r-(trq_dem_l-trq_dem_lm-trq_dem_lr))));
    end
    bra_pre_l=single(0);
    bra_pre_r=single(0);
    mode=int8(34);
elseif guzhang_lf==0 && guzhang_lm==1 && guzhang_lr==0 && guzhang_rf==1 && guzhang_rm==1 && guzhang_rr==0    %3电机故障，同侧电机进行力矩转移，超过限值后，对侧亦降扭。  右前-右中-左中 对侧
    trq_dem_rf=single(0);
    trq_dem_rm=single(0);
    trq_dem_lm=single(0);
    trq_dem_rr=single(min(trq_dem_r,trqlim_rr));
    trq_dem_lf=single(min(trq_dem_l/2,trqlim_lf));
    trq_dem_lr=single(min(trq_dem_l/2,trqlim_lr));
    if (trq_dem_r-trq_dem_rr)>=(trq_dem_l-trq_dem_lf-trq_dem_lr)
        trq_dem_lf=single(min(trqlim_lf,(trq_dem_l-(trq_dem_r-trq_dem_rr))/2));
        trq_dem_lr=single(min(trqlim_lr,(trq_dem_l-(trq_dem_r-trq_dem_rr))/2));
    else
        trq_dem_rr=single(min(trqlim_rr,(trq_dem_r-(trq_dem_l-trq_dem_lf-trq_dem_lr))));
    end
    bra_pre_l=single(0);
    bra_pre_r=single(0);
    mode=int8(35);
elseif guzhang_lf==0 && guzhang_lm==0 && guzhang_lr==1 && guzhang_rf==1 && guzhang_rm==1 && guzhang_rr==0    %3电机故障，同侧电机进行力矩转移，超过限值后，对侧亦降扭。  右前-右中-左后 对侧
    trq_dem_rf=single(0);
    trq_dem_rm=single(0);
    trq_dem_lr=single(0);
    trq_dem_rr=single(min(trq_dem_r,trqlim_rr));
    trq_dem_lf=single(min(trq_dem_l/2,trqlim_lf));
    trq_dem_lm=single(min(trq_dem_l/2,trqlim_lm));
    if (trq_dem_r-trq_dem_rr)>=(trq_dem_l-trq_dem_lf-trq_dem_lm)
        trq_dem_lf=single(min(trqlim_lf,(trq_dem_l-(trq_dem_r-trq_dem_rr))/2));
        trq_dem_lm=single(min(trqlim_lm,(trq_dem_l-(trq_dem_r-trq_dem_rr))/2));
    else
        trq_dem_rr=single(min(trqlim_rr,(trq_dem_r-(trq_dem_l-trq_dem_lf-trq_dem_lm))));
    end
    bra_pre_l=single(0);
    bra_pre_r=single(0);
    mode=int8(36);
    
elseif guzhang_lf==1 && guzhang_lm==0 && guzhang_lr==0 && guzhang_rf==1 && guzhang_rm==0 && guzhang_rr==1    %3电机故障，同侧电机进行力矩转移，超过限值后，对侧亦降扭。  右前-右后-左前 对侧
    trq_dem_rf=single(0);
    trq_dem_rr=single(0);
    trq_dem_lf=single(0);
    trq_dem_rm=single(min(trq_dem_r,trqlim_rm));
    trq_dem_lm=single(min(trq_dem_l/2,trqlim_lm));
    trq_dem_lr=single(min(trq_dem_l/2,trqlim_lr));
    if (trq_dem_r-trq_dem_rm)>=(trq_dem_l-trq_dem_lm-trq_dem_lr)
        trq_dem_lm=single(min(trqlim_lm,(trq_dem_l-(trq_dem_r-trq_dem_rm))/2));
        trq_dem_lr=single(min(trqlim_lr,(trq_dem_l-(trq_dem_r-trq_dem_rm))/2));
    else
        trq_dem_rm=single(min(trqlim_rm,(trq_dem_r-(trq_dem_l-trq_dem_lm-trq_dem_lr))));
    end
    bra_pre_l=single(0);
    bra_pre_r=single(0);
    mode=int8(37);
elseif guzhang_lf==0 && guzhang_lm==1 && guzhang_lr==0 && guzhang_rf==1 && guzhang_rm==0 && guzhang_rr==1    %3电机故障，同侧电机进行力矩转移，超过限值后，对侧亦降扭。  右前-右后-左中 对侧
    trq_dem_rf=single(0);
    trq_dem_rr=single(0);
    trq_dem_lm=single(0);
    trq_dem_rm=single(min(trq_dem_r,trqlim_rm));
    trq_dem_lf=single(min(trq_dem_l/2,trqlim_lf));
    trq_dem_lr=single(min(trq_dem_l/2,trqlim_lr));
    if (trq_dem_r-trq_dem_rm)>=(trq_dem_l-trq_dem_lf-trq_dem_lr)
        trq_dem_lf=single(min(trqlim_lf,(trq_dem_l-(trq_dem_r-trq_dem_rm))/2));
        trq_dem_lr=single(min(trqlim_lr,(trq_dem_l-(trq_dem_r-trq_dem_rm))/2));
    else
        trq_dem_rm=single(min(trqlim_rm,(trq_dem_r-(trq_dem_l-trq_dem_lf-trq_dem_lr))));
    end
    bra_pre_l=single(0);
    bra_pre_r=single(0);
    mode=int8(38);
elseif guzhang_lf==0 && guzhang_lm==0 && guzhang_lr==1 && guzhang_rf==1 && guzhang_rm==0 && guzhang_rr==1    %3电机故障，同侧电机进行力矩转移，超过限值后，对侧亦降扭。  右前-右后-左后 对侧
    trq_dem_rf=single(0);
    trq_dem_rr=single(0);
    trq_dem_lr=single(0);
    trq_dem_rm=single(min(trq_dem_r,trqlim_rm));
    trq_dem_lf=single(min(trq_dem_l/2,trqlim_lf));
    trq_dem_lm=single(min(trq_dem_l/2,trqlim_lm));
    if (trq_dem_r-trq_dem_rm)>=(trq_dem_l-trq_dem_lf-trq_dem_lm)
        trq_dem_lf=single(min(trqlim_lf,(trq_dem_l-(trq_dem_r-trq_dem_rm))/2));
        trq_dem_lm=single(min(trqlim_lm,(trq_dem_l-(trq_dem_r-trq_dem_rm))/2));
    else
        trq_dem_rm=single(min(trqlim_rm,(trq_dem_r-(trq_dem_l-trq_dem_lf-trq_dem_lm))));
    end
    bra_pre_l=single(0);
    bra_pre_r=single(0);
    mode=int8(39);
    
elseif guzhang_lf==1 && guzhang_lm==0 && guzhang_lr==0 && guzhang_rf==0 && guzhang_rm==1 && guzhang_rr==1    %3电机故障，同侧电机进行力矩转移，超过限值后，对侧亦降扭。  右中-右后-左前 对侧
    trq_dem_rm=single(0);
    trq_dem_rr=single(0);
    trq_dem_lf=single(0);
    trq_dem_rf=single(min(trq_dem_r,trqlim_rf));
    trq_dem_lm=single(min(trq_dem_l/2,trqlim_lm));
    trq_dem_lr=single(min(trq_dem_l/2,trqlim_lr));
    if (trq_dem_r-trq_dem_rf)>=(trq_dem_l-trq_dem_lm-trq_dem_lr)
        trq_dem_lm=single(min(trqlim_lm,(trq_dem_l-(trq_dem_r-trq_dem_rf))/2));
        trq_dem_lr=single(min(trqlim_lr,(trq_dem_l-(trq_dem_r-trq_dem_rf))/2));
    else
        trq_dem_rf=single(min(trqlim_rf,(trq_dem_r-(trq_dem_l-trq_dem_lm-trq_dem_lr))));
    end
    bra_pre_l=single(0);
    bra_pre_r=single(0);
    mode=int8(40);
elseif guzhang_lf==0 && guzhang_lm==1 && guzhang_lr==0 && guzhang_rf==0 && guzhang_rm==1 && guzhang_rr==1    %3电机故障，同侧电机进行力矩转移，超过限值后，对侧亦降扭。  右中-右后-左中 对侧
    trq_dem_rm=single(0);
    trq_dem_rr=single(0);
    trq_dem_lm=single(0);
    trq_dem_rf=single(min(trq_dem_r,trqlim_rf));
    trq_dem_lf=single(min(trq_dem_l/2,trqlim_lf));
    trq_dem_lr=single(min(trq_dem_l/2,trqlim_lr));
    if (trq_dem_r-trq_dem_rf)>=(trq_dem_l-trq_dem_lf-trq_dem_lr)
        trq_dem_lf=single(min(trqlim_lf,(trq_dem_l-(trq_dem_r-trq_dem_rf))/2));
        trq_dem_lr=single(min(trqlim_lr,(trq_dem_l-(trq_dem_r-trq_dem_rf))/2));
    else
        trq_dem_rf=single(min(trqlim_rf,(trq_dem_r-(trq_dem_l-trq_dem_lf-trq_dem_lr))));
    end
    bra_pre_l=single(0);
    bra_pre_r=single(0);
    mode=int8(41);
elseif guzhang_lf==0 && guzhang_lm==0 && guzhang_lr==1 && guzhang_rf==0 && guzhang_rm==1 && guzhang_rr==1    %3电机故障，同侧电机进行力矩转移，超过限值后，对侧亦降扭。  右中-右后-左后 对侧
    trq_dem_rm=single(0);
    trq_dem_rr=single(0);
    trq_dem_lr=single(0);
    trq_dem_rf=single(min(trq_dem_r,trqlim_rf));
    trq_dem_lf=single(min(trq_dem_l/2,trqlim_lf));
    trq_dem_lm=single(min(trq_dem_l/2,trqlim_lm));
    if (trq_dem_r-trq_dem_rf)>=(trq_dem_l-trq_dem_lf-trq_dem_lm)
        trq_dem_lf=single(min(trqlim_lf,(trq_dem_l-(trq_dem_r-trq_dem_rf))/2));
        trq_dem_lm=single(min(trqlim_lm,(trq_dem_l-(trq_dem_r-trq_dem_rf))/2));
    else
        trq_dem_rf=single(min(trqlim_rf,(trq_dem_r-(trq_dem_l-trq_dem_lf-trq_dem_lm))));
    end
    bra_pre_l=single(0);
    bra_pre_r=single(0);
    mode=int8(42);
    
    
    
    
    
    
    
    
    
    
    
    
    
    
elseif (guzhang_lf==1 && guzhang_lm==1 && guzhang_lr==1 && guzhang_rf==1 && guzhang_rm==0 && guzhang_rr==0) || (guzhang_lf==1 && guzhang_lm==1 && guzhang_lr==1 && guzhang_rf==0 && guzhang_rm==1 && guzhang_rr==0) || (guzhang_lf==1 && guzhang_lm==1 && guzhang_lr==1 && guzhang_rf==0 && guzhang_rm==0 && guzhang_rr==1)    %4电机故障，同侧电机进行力矩转移，超过限值后，对侧亦降扭。  左前 左中 左后 右前/右中/右后   左侧
    trq_dem_lf=single(0);
    trq_dem_lm=single(0);
    trq_dem_lr=single(0);
    trq_dem_rf=single(0);
    trq_dem_rm=single(0);
    trq_dem_rr=single(0);
    bra_pre_l=single(bra_pre_gz2);
    bra_pre_r=single(bra_pre_gz2);
    mode=int8(43);
elseif (guzhang_lf==1 && guzhang_lm==0 && guzhang_lr==0 && guzhang_rf==1 && guzhang_rm==1 && guzhang_rr==1) || (guzhang_lf==0 && guzhang_lm==1 && guzhang_lr==0 && guzhang_rf==1 && guzhang_rm==1 && guzhang_rr==1) || (guzhang_lf==0 && guzhang_lm==0 && guzhang_lr==1 && guzhang_rf==1 && guzhang_rm==1 && guzhang_rr==1)   %4电机故障，同侧电机进行力矩转移，超过限值后，对侧亦降扭。  右前 右中 右后 左前/左中/左后   右侧
    trq_dem_lf=single(0);
    trq_dem_lm=single(0);
    trq_dem_lr=single(0);
    trq_dem_rf=single(0);
    trq_dem_rm=single(0);
    trq_dem_rr=single(0);
    bra_pre_l=single(bra_pre_gz2);
    bra_pre_r=single(bra_pre_gz2);
    mode=int8(44);
    
elseif guzhang_lf==1 && guzhang_lm==1 && guzhang_lr==0 && guzhang_rf==1 && guzhang_rm==1 && guzhang_rr==0    %4电机故障，同侧电机进行力矩转移，超过限值后，对侧亦降扭。  左前-左中-右前-右中 对侧
    trq_dem_lf=single(0);
    trq_dem_lm=single(0);
    trq_dem_rf=single(0);
    trq_dem_rm=single(0);
    trq_dem_lr=single(min(trq_dem_l,trqlim_lr));
    trq_dem_rr=single(min(trq_dem_r,trqlim_rr));
    if (trq_dem_l-trq_dem_lr)>=(trq_dem_r-trq_dem_rr)
        trq_dem_rr=single(min(trqlim_rr,(trq_dem_r-(trq_dem_l-trq_dem_lr))));
    else
        trq_dem_lr=single(min(trqlim_lr,(trq_dem_l-(trq_dem_r-trq_dem_rr))));
    end
    bra_pre_l=single(0);
    bra_pre_r=single(0);
    mode=int8(45);
elseif guzhang_lf==1 && guzhang_lm==1 && guzhang_lr==0 && guzhang_rf==1 && guzhang_rm==0 && guzhang_rr==1    %4电机故障，同侧电机进行力矩转移，超过限值后，对侧亦降扭。  左前-左中-右前-右后 对侧
    trq_dem_lf=single(0);
    trq_dem_lm=single(0);
    trq_dem_rf=single(0);
    trq_dem_rr=single(0);
    trq_dem_lr=single(min(trq_dem_l,trqlim_lr));
    trq_dem_rm=single(min(trq_dem_r,trqlim_rm));
    if (trq_dem_l-trq_dem_lr)>=(trq_dem_r-trq_dem_rm)
        trq_dem_rm=single(min(trqlim_rm,(trq_dem_r-(trq_dem_l-trq_dem_lr))));
    else
        trq_dem_lr=single(min(trqlim_lr,(trq_dem_l-(trq_dem_r-trq_dem_rm))));
    end
    bra_pre_l=single(0);
    bra_pre_r=single(0);
    mode=int8(46);
elseif guzhang_lf==1 && guzhang_lm==1 && guzhang_lr==0 && guzhang_rf==0 && guzhang_rm==1 && guzhang_rr==1    %4电机故障，同侧电机进行力矩转移，超过限值后，对侧亦降扭。  左前-左中-右中-右后 对侧
    trq_dem_lf=single(0);
    trq_dem_lm=single(0);
    trq_dem_rm=single(0);
    trq_dem_rr=single(0);
    trq_dem_lr=single(min(trq_dem_l,trqlim_lr));
    trq_dem_rf=single(min(trq_dem_r,trqlim_rf));
    if (trq_dem_l-trq_dem_lr)>=(trq_dem_r-trq_dem_rf)
        trq_dem_rf=single(min(trqlim_rf,(trq_dem_r-(trq_dem_l-trq_dem_lr))));
    else
        trq_dem_lr=single(min(trqlim_lr,(trq_dem_l-(trq_dem_r-trq_dem_rf))));
    end
    bra_pre_l=single(0);
    bra_pre_r=single(0);
    mode=int8(47);
    
elseif guzhang_lf==1 && guzhang_lm==0 && guzhang_lr==1 && guzhang_rf==1 && guzhang_rm==1 && guzhang_rr==0    %4电机故障，同侧电机进行力矩转移，超过限值后，对侧亦降扭。  左前-左后-右前-右中 对侧
    trq_dem_lf=single(0);
    trq_dem_lr=single(0);
    trq_dem_rf=single(0);
    trq_dem_rm=single(0);
    trq_dem_lm=single(min(trq_dem_l,trqlim_lm));
    trq_dem_rr=single(min(trq_dem_r,trqlim_rr));
    if (trq_dem_l-trq_dem_lm)>=(trq_dem_r-trq_dem_rr)
        trq_dem_rr=single(min(trqlim_rr,(trq_dem_r-(trq_dem_l-trq_dem_lm))));
    else
        trq_dem_lm=single(min(trqlim_lm,(trq_dem_l-(trq_dem_r-trq_dem_rr))));
    end
    bra_pre_l=single(0);
    bra_pre_r=single(0);
    mode=int8(48);
elseif guzhang_lf==1 && guzhang_lm==0 && guzhang_lr==1 && guzhang_rf==1 && guzhang_rm==0 && guzhang_rr==1    %4电机故障，同侧电机进行力矩转移，超过限值后，对侧亦降扭。  左前-左后-右前-右后 对侧
    trq_dem_lf=single(0);
    trq_dem_lr=single(0);
    trq_dem_rf=single(0);
    trq_dem_rr=single(0);
    trq_dem_lm=single(min(trq_dem_l,trqlim_lm));
    trq_dem_rm=single(min(trq_dem_r,trqlim_rm));
    if (trq_dem_l-trq_dem_lm)>=(trq_dem_r-trq_dem_rm)
        trq_dem_rm=single(min(trqlim_rm,(trq_dem_r-(trq_dem_l-trq_dem_lm))));
    else
        trq_dem_lm=single(min(trqlim_lm,(trq_dem_l-(trq_dem_r-trq_dem_rm))));
    end
    bra_pre_l=single(0);
    bra_pre_r=single(0);
    mode=int8(49);
elseif guzhang_lf==1 && guzhang_lm==0 && guzhang_lr==1 && guzhang_rf==0 && guzhang_rm==1 && guzhang_rr==1    %4电机故障，同侧电机进行力矩转移，超过限值后，对侧亦降扭。  左前-左后-右中-右后 对侧
    trq_dem_lf=single(0);
    trq_dem_lr=single(0);
    trq_dem_rm=single(0);
    trq_dem_rr=single(0);
    trq_dem_lm=single(min(trq_dem_l,trqlim_lm));
    trq_dem_rf=single(min(trq_dem_r,trqlim_rf));
    if (trq_dem_l-trq_dem_lm)>=(trq_dem_r-trq_dem_rf)
        trq_dem_rf=single(min(trqlim_rf,(trq_dem_r-(trq_dem_l-trq_dem_lm))));
    else
        trq_dem_lm=single(min(trqlim_lm,(trq_dem_l-(trq_dem_r-trq_dem_rf))));
    end
    bra_pre_l=single(0);
    bra_pre_r=single(0);
    mode=int8(50);
    
elseif guzhang_lf==0 && guzhang_lm==1 && guzhang_lr==1 && guzhang_rf==1 && guzhang_rm==1 && guzhang_rr==0    %4电机故障，同侧电机进行力矩转移，超过限值后，对侧亦降扭。  左中-左后-右前-右中 对侧
    trq_dem_lm=single(0);
    trq_dem_lr=single(0);
    trq_dem_rf=single(0);
    trq_dem_rm=single(0);
    trq_dem_lf=single(min(trq_dem_l,trqlim_lf));
    trq_dem_rr=single(min(trq_dem_r,trqlim_rr));
    if (trq_dem_l-trq_dem_lf)>=(trq_dem_r-trq_dem_rr)
        trq_dem_rr=single(min(trqlim_rr,(trq_dem_r-(trq_dem_l-trq_dem_lf))));
    else
        trq_dem_lf=single(min(trqlim_lf,(trq_dem_l-(trq_dem_r-trq_dem_rr))));
    end
    bra_pre_l=single(0);
    bra_pre_r=single(0);
    mode=int8(51);
elseif guzhang_lf==0 && guzhang_lm==1 && guzhang_lr==1 && guzhang_rf==1 && guzhang_rm==0 && guzhang_rr==1    %4电机故障，同侧电机进行力矩转移，超过限值后，对侧亦降扭。  左中-左后-右前-右后 对侧
    trq_dem_lm=single(0);
    trq_dem_lr=single(0);
    trq_dem_rf=single(0);
    trq_dem_rr=single(0);
    trq_dem_lf=single(min(trq_dem_l,trqlim_lf));
    trq_dem_rm=single(min(trq_dem_r,trqlim_rm));
    if (trq_dem_l-trq_dem_lf)>=(trq_dem_r-trq_dem_rm)
        trq_dem_rm=single(min(trqlim_rm,(trq_dem_r-(trq_dem_l-trq_dem_lf))));
    else
        trq_dem_lf=single(min(trqlim_lf,(trq_dem_l-(trq_dem_r-trq_dem_rm))));
    end
    bra_pre_l=single(0);
    bra_pre_r=single(0);
    mode=int8(52);
elseif guzhang_lf==0 && guzhang_lm==1 && guzhang_lr==1 && guzhang_rf==0 && guzhang_rm==1 && guzhang_rr==1    %4电机故障，同侧电机进行力矩转移，超过限值后，对侧亦降扭。  左中-左后-右中-右后 对侧
    trq_dem_lm=single(0);
    trq_dem_lr=single(0);
    trq_dem_rm=single(0);
    trq_dem_rr=single(0);
    trq_dem_lf=single(min(trq_dem_l,trqlim_lf));
    trq_dem_rf=single(min(trq_dem_r,trqlim_rf));
    if (trq_dem_l-trq_dem_lf)>=(trq_dem_r-trq_dem_rf)
        trq_dem_rf=single(min(trqlim_rf,(trq_dem_r-(trq_dem_l-trq_dem_lf))));
    else
        trq_dem_lf=single(min(trqlim_lf,(trq_dem_l-(trq_dem_r-trq_dem_rf))));
    end
    bra_pre_l=single(0);
    bra_pre_r=single(0);
    mode=int8(53);
    
    
    
    
    
    
    
    
    
    
    
    
elseif (guzhang_lf==0 && guzhang_lm==1 && guzhang_lr==1 && guzhang_rf==1 && guzhang_rm==1 && guzhang_rr==1) || (guzhang_lf==1 && guzhang_lm==0 && guzhang_lr==1 && guzhang_rf==1 && guzhang_rm==1 && guzhang_rr==1) || (guzhang_lf==1 && guzhang_lm==1 && guzhang_lr==0 && guzhang_rf==1 && guzhang_rm==1 && guzhang_rr==1) || (guzhang_lf==1 && guzhang_lm==1 && guzhang_lr==1 && guzhang_rf==0 && guzhang_rm==1 && guzhang_rr==1) || (guzhang_lf==1 && guzhang_lm==1 && guzhang_lr==1 && guzhang_rf==1 && guzhang_rm==0 && guzhang_rr==1) || (guzhang_lf==1 && guzhang_lm==1 && guzhang_lr==1 && guzhang_rf==1 && guzhang_rm==1 && guzhang_rr==0)  %5电机故障，同侧电机进行力矩转移，超过限值后，对侧亦降扭。  左前 左中 左后 右前/右中/右后   左侧
    trq_dem_lf=single(0);
    trq_dem_lm=single(0);
    trq_dem_lr=single(0);
    trq_dem_rf=single(0);
    trq_dem_rm=single(0);
    trq_dem_rr=single(0);
    bra_pre_l=single(bra_pre_gz2);
    bra_pre_r=single(bra_pre_gz2);
    mode=int8(54);
    
    
    
    
    
    
    
else    %6电机故障，同侧电机进行力矩转移，超过限值后，对侧亦降扭。  左前 左中 左后 右前/右中/右后   左侧
    trq_dem_lf=single(0);
    trq_dem_lm=single(0);
    trq_dem_lr=single(0);
    trq_dem_rf=single(0);
    trq_dem_rm=single(0);
    trq_dem_rr=single(0);
    bra_pre_l=single(bra_pre_gz2);
    bra_pre_r=single(bra_pre_gz2);
    mode=int8(55);
end
    
    
    
    
    
    
    
    % trq_dem_lf=max(0,trq_dem_lf);%电机转矩不小于0，就是不能出现负值
    % trq_dem_lr=max(0,trq_dem_lr);
    % trq_dem_rf=max(0,trq_dem_rf);
    % trq_dem_rr=max(0,trq_dem_rr);
    trq_dem_lf=single(max(-trqlim_lf,trq_dem_lf));%电机转矩可以出现负值，不超过负的外特性
    trq_dem_lm=single(max(-trqlim_lm,trq_dem_lm));
    trq_dem_lr=single(max(-trqlim_lr,trq_dem_lr));
    trq_dem_rf=single(max(-trqlim_rf,trq_dem_rf));
    trq_dem_rm=single(max(-trqlim_rm,trq_dem_rm));
    trq_dem_rr=single(max(-trqlim_rr,trq_dem_rr));
    bra_pre_l=single(bra_pre_l);
    bra_pre_r=single(bra_pre_r);
end

== system six_plus_six_AcmsteeringV09_main/MainControl/mode_control/forward/forward/Drive/容错控制 ==
  trq_dem_l : Inport
  trq_dem_r : Inport  Port=2
  trqlim_lf : Inport  Port=3
  trqlim_lm : Inport  Port=4
  trqlim_lr : Inport  Port=5
  trqlim_rf : Inport  Port=6
  trqlim_rm : Inport  Port=7
  trqlim_rr : Inport  Port=8
  guzhang_lf : Inport  Port=9
  guzhang_lm : Inport  Port=10
  guzhang_lr : Inport  Port=11
  guzhang_rf : Inport  Port=12
  guzhang_rm : Inport  Port=13
  guzhang_rr : Inport  Port=14
  Constant : Constant  Value=bra_pre_gz2  OutDataTypeStr=single  SampleTime=-1
  Constant1 : Constant  Value=bra_pre_gz34  OutDataTypeStr=single  SampleTime=-1
  Constant11 : Constant  Value=RC_switch  OutDataTypeStr=single  SampleTime=-1
  Data Type Conversion{,1..5} (6 alike) : DataTypeConversion
  ECCalVar : Constant  InitFcn=ecucoder_acal;  Value=guzhang_lf  OutDataTypeStr=Inherit: Inherit via back propagation  SampleTime=-1
  ECCalVar1 : Constant  InitFcn=ecucoder_acal;  Value=guzhang_lm  OutDataTypeStr=Inherit: Inherit via back propagation  SampleTime=-1
  ECCalVar2 : Constant  InitFcn=ecucoder_acal;  Value=guzhang_lr  OutDataTypeStr=Inherit: Inherit via back propagation  SampleTime=-1
  ECCalVar3 : Constant  InitFcn=ecucoder_acal;  Value=guzhang_rf  OutDataTypeStr=Inherit: Inherit via back propagation  SampleTime=-1
  ECCalVar4 : Constant  InitFcn=ecucoder_acal;  Value=guzhang_rm  OutDataTypeStr=Inherit: Inherit via back propagation  SampleTime=-1
  ECCalVar5 : Constant  InitFcn=ecucoder_acal;  Value=guzhang_rr  OutDataTypeStr=Inherit: Inherit via back propagation  SampleTime=-1
  MATLAB Function : MATLAB Function  TreatAsAtomicUnit=on
  MATLAB Function5 : MATLAB Function  TreatAsAtomicUnit=on
  Terminator : Terminator
  trq_dem_lf : Outport
  trq_dem_lm : Outport  Port=2
  trq_dem_lr : Outport  Port=3
  trq_dem_rf : Outport  Port=4
  trq_dem_rm : Outport  Port=5
  trq_dem_rr : Outport  Port=6
  bra_pre_l : Outport  Port=7
  bra_pre_r : Outport  Port=8
  wires:
  trq_dem_r/1 -> MATLAB Function/2(trq_dem_r)
  trqlim_lr/1 -> MATLAB Function/5(trqlim_lr)
  trq_dem_l/1 -> MATLAB Function/1(trq_dem_l)
  trqlim_rf/1 -> MATLAB Function/6(trqlim_rf)
  trqlim_rr/1 -> MATLAB Function/8(trqlim_rr)
  trqlim_lf/1 -> MATLAB Function/3(trqlim_lf)
  MATLAB Function/1(trq_dem_lf) -> trq_dem_lf/1
  MATLAB Function/3(trq_dem_lr) -> trq_dem_lr/1
  MATLAB Function/4(trq_dem_rf) -> trq_dem_rf/1
  MATLAB Function/6(trq_dem_rr) -> trq_dem_rr/1
  MATLAB Function/7(bra_pre_l) -> bra_pre_l/1
  MATLAB Function/8(bra_pre_r) -> bra_pre_r/1
  Constant/1 -> MATLAB Function/15(bra_pre_gz2)
  Constant1/1 -> MATLAB Function/16(bra_pre_gz34)
  MATLAB Function/9(mode) -> Terminator/1
  trqlim_lm/1 -> MATLAB Function/4(trqlim_lm)
  trqlim_rm/1 -> MATLAB Function/7(trqlim_rm)
  MATLAB Function/2(trq_dem_lm) -> trq_dem_lm/1
  MATLAB Function/5(trq_dem_rm) -> trq_dem_rm/1
  Constant11/1 -> MATLAB Function5/1(RC_switch)
  MATLAB Function5/1(guzhang_lf1) -> Data Type Conversion/1
  MATLAB Function5/2(guzhang_lm1) -> Data Type Conversion1/1
  MATLAB Function5/3(guzhang_lr1) -> Data Type Conversion2/1
  MATLAB Function5/4(guzhang_rf1) -> Data Type Conversion3/1
  MATLAB Function5/6(guzhang_rr1) -> Data Type Conversion5/1
  MATLAB Function5/5(guzhang_rm1) -> Data Type Conversion4/1
  ECCalVar/1 -> MATLAB Function5/2(guzhang_lf)
  ECCalVar1/1 -> MATLAB Function5/3(guzhang_lm)
  ECCalVar2/1 -> MATLAB Function5/4(guzhang_lr)
  ECCalVar3/1 -> MATLAB Function5/5(guzhang_rf)
  ECCalVar4/1 -> MATLAB Function5/6(guzhang_rm)
  ECCalVar5/1 -> MATLAB Function5/7(guzhang_rr)
  Data Type Conversion/1 -> MATLAB Function/9(guzhang_lf)  "guzhang_lf"
  Data Type Conversion1/1 -> MATLAB Function/10(guzhang_lm)  "guzhang_lm"
  Data Type Conversion2/1 -> MATLAB Function/11(guzhang_lr)  "guzhang_lr"
  Data Type Conversion3/1 -> MATLAB Function/12(guzhang_rf)  "guzhang_rf"
  Data Type Conversion4/1 -> MATLAB Function/13(guzhang_rm)  "guzhang_rm"
  Data Type Conversion5/1 -> MATLAB Function/14(guzhang_rr)  "guzhang_rr"
